simulink model "k1modalprm"  (Simulink 8.6)
settings: Solver=VariableStepAuto  StartTime=0.0  StopTime=10.0  RelTol=1e-3
libraries: cdsIPCx x18, cdsAdcx0 x1, VISMODAL_MASTER x1, cdsParameters x1
settings Model: Creator=controls  LastModifiedBy=controls
settings DataIOCC: SaveFormat=Dataset  SignalLoggingSaveFormat=Dataset
settings OptimizationCC: ExpressionDepthLimit=128
settings DebuggingCC: UnderspecifiedInitializationDetection=Simplified  MergeDetectMultiDrivingBlocksExec=error  SolverPrmCheckMsg=none  FcnCallInpInsideContextMsg=EnableAllAsError  StateNameClashWarn=none
settings HardwareCC: ProdBitPerPointer=64  ProdLargestAtomicFloat=Float  ProdIntDivRoundTo=Zero  ProdEndianess=LittleEndian  ProdWordSize=64  ProdHWDeviceType=Intel->x86-64 (Windows64)
settings GRTTargetCC: GeneratePreprocessorConditionals=Use local settings  CombineOutputUpdateFcns=on  GRTInterface=off
settings ConfigComp: CovModelRefEnable=off

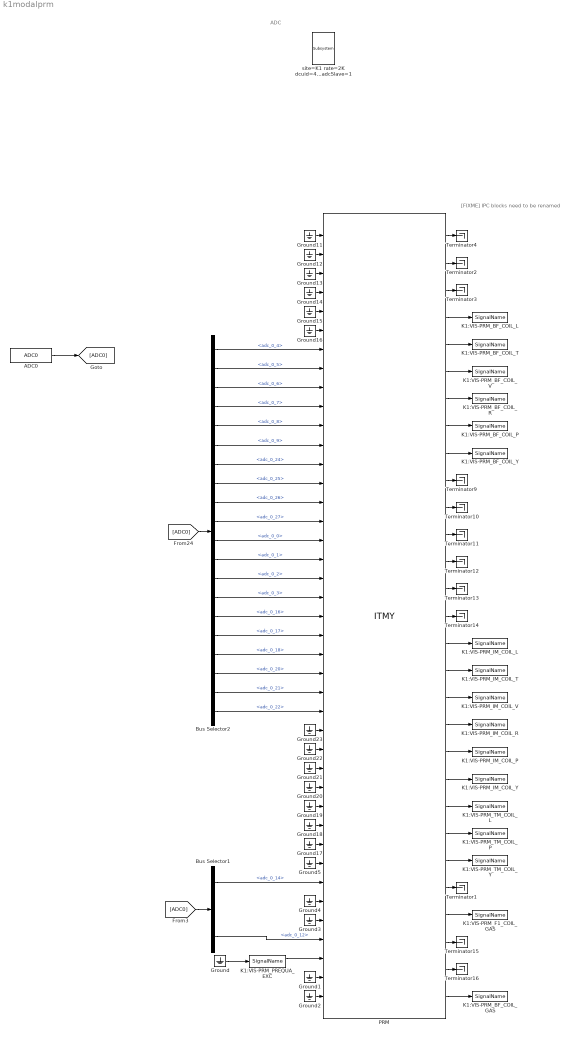
== system k1modalprm ==
  note: ADC
  note: [FIXME] IPC blocks need to be renamed
  ADC0 : cdsAdcx0/ADC0  Tag=cdsAdc  Description=|
      | type-GSC_16AI64SSA
      | card_num=0
      settings: AttributesFormatString=%<Description>\n%<Tag>
  Bus Selector1 : BusSelector  Description=ADC Selector  OutputSignals=adc_0_14,adc_0_13,adc_0_12
      settings: AttributesFormatString=%<Description>
  Bus Selector2 : BusSelector  Description=ADC Selector  OutputSignals=adc_0_4,adc_0_5,adc_0_6,adc_0_7,adc_0_8,adc_0_9,adc_0_24,adc_0_25,adc_0_26,adc_0_27,adc_0_0,adc_0_1,adc_0_2,adc_0_3,adc_0_16,adc_0_17,adc_0_18,adc_0_20,adc_0_21,adc_0_22
      settings: AttributesFormatString=%<Description>
  Ground{,1..5,11..23} (19 alike) : Ground
  K1:VIS-PRM_BF_COIL_GAS : cdsIPCx/SignalName  Tag=cdsIPCx_SHMEM  Description=Inter-Process Communication via Shared memory.
      settings: AttributesFormatString=%<Tag>
  K1:VIS-PRM_BF_COIL_L : cdsIPCx/SignalName  Tag=cdsIPCx_SHMEM  Description=Inter-Process Communication via Shared memory.
      settings: AttributesFormatString=%<Tag>
  K1:VIS-PRM_BF_COIL_P : cdsIPCx/SignalName  Tag=cdsIPCx_SHMEM  Description=Inter-Process Communication via Shared memory.
      settings: AttributesFormatString=%<Tag>
  K1:VIS-PRM_BF_COIL_R : cdsIPCx/SignalName  Tag=cdsIPCx_SHMEM  Description=Inter-Process Communication via Shared memory.
      settings: AttributesFormatString=%<Tag>
  K1:VIS-PRM_BF_COIL_T : cdsIPCx/SignalName  Tag=cdsIPCx_SHMEM  Description=Inter-Process Communication via Shared memory.
      settings: AttributesFormatString=%<Tag>
  K1:VIS-PRM_BF_COIL_V : cdsIPCx/SignalName  Tag=cdsIPCx_SHMEM  Description=Inter-Process Communication via Shared memory.
      settings: AttributesFormatString=%<Tag>
  K1:VIS-PRM_BF_COIL_Y : cdsIPCx/SignalName  Tag=cdsIPCx_SHMEM  Description=Inter-Process Communication via Shared memory.
      settings: AttributesFormatString=%<Tag>
  K1:VIS-PRM_F1_COIL_GAS : cdsIPCx/SignalName  Tag=cdsIPCx_SHMEM  Description=Inter-Process Communication via Shared memory.
      settings: AttributesFormatString=%<Tag>
  K1:VIS-PRM_IM_COIL_L : cdsIPCx/SignalName  Tag=cdsIPCx_SHMEM  Description=Inter-Process Communication via Shared memory.
      settings: AttributesFormatString=%<Tag>
  K1:VIS-PRM_IM_COIL_P : cdsIPCx/SignalName  Tag=cdsIPCx_SHMEM  Description=Inter-Process Communication via Shared memory.
      settings: AttributesFormatString=%<Tag>
  K1:VIS-PRM_IM_COIL_R : cdsIPCx/SignalName  Tag=cdsIPCx_SHMEM  Description=Inter-Process Communication via Shared memory.
      settings: AttributesFormatString=%<Tag>
  K1:VIS-PRM_IM_COIL_T : cdsIPCx/SignalName  Tag=cdsIPCx_SHMEM  Description=Inter-Process Communication via Shared memory.
      settings: AttributesFormatString=%<Tag>
  K1:VIS-PRM_IM_COIL_V : cdsIPCx/SignalName  Tag=cdsIPCx_SHMEM  Description=Inter-Process Communication via Shared memory.
      settings: AttributesFormatString=%<Tag>
  K1:VIS-PRM_IM_COIL_Y : cdsIPCx/SignalName  Tag=cdsIPCx_SHMEM  Description=Inter-Process Communication via Shared memory.
      settings: AttributesFormatString=%<Tag>
  K1:VIS-PRM_PREQUA_EXC : cdsIPCx/SignalName  Tag=cdsIPCx_SHMEM  Description=Inter-Process Communication via Shared memory.
      settings: AttributesFormatString=%<Tag>
  K1:VIS-PRM_TM_COIL_L : cdsIPCx/SignalName  Tag=cdsIPCx_SHMEM  Description=Inter-Process Communication via Shared memory.
      settings: AttributesFormatString=%<Tag>
  K1:VIS-PRM_TM_COIL_P : cdsIPCx/SignalName  Tag=cdsIPCx_SHMEM  Description=Inter-Process Communication via Shared memory.
      settings: AttributesFormatString=%<Tag>
  K1:VIS-PRM_TM_COIL_Y : cdsIPCx/SignalName  Tag=cdsIPCx_SHMEM  Description=Inter-Process Communication via Shared memory.
      settings: AttributesFormatString=%<Tag>
  PRM : VISMODAL_MASTER/ITMY
  Terminator{1..4,9..16} (12 alike) : Terminator
  site=K1 rate=2K dcuid=45 host=k1prm specific_cpu=3 adcSlave=1 : cdsParameters/Subsystem  Tag=cdsParameters  Description=|
      | Purpose:                                                                                                                                                                                                                                
      | Provide system parameters to the FE code generator to properly configure the generated EPICS names, rep rate of the FE controller, and the Data Acquisition node ID for proper storage of data from this FE controller.                 
      |                                                                                                                                                                                                                                         
      | Useage:                                                                                                                                                                                                                                 
      | The part NAME field is used to identify the FE parameters. It must be of the form:                                                                                                                                                      
      | site=                                                                                                                                                                                                                                   
      | rate=                                                                                                                                                                                                                                   
      | dcuid=                                                                                                                                                                                                                                  
      |                                                                                                                                                                                                                                         
      | Where:                                                                                                                                                                                                                                  
      | site= argument may be H1, H2, L1, M1, G1, either as a single argument or multiple, for example site=H1,H2. These are the only names allowed. These will become the first two characters of all EPICS and signal names (for example G1:).
      |                                                                                                                                                                                                                                         
      | rate= may be 2K, 16K, 32K, or 64K                                                                                                                                                                                                       
      |                                                                                                                                                                                                                                         
      | dcuid= is site specific ie it must be unique at each site.
      settings: AttributesFormatString=%<Tag>
  wires:
  PRM/16 -> K1:VIS-PRM_IM_COIL_L/1
  PRM/17 -> K1:VIS-PRM_IM_COIL_T/1
  PRM/18 -> K1:VIS-PRM_IM_COIL_V/1
  PRM/19 -> K1:VIS-PRM_IM_COIL_R/1
  PRM/20 -> K1:VIS-PRM_IM_COIL_P/1
  PRM/21 -> K1:VIS-PRM_IM_COIL_Y/1
  PRM/22 -> K1:VIS-PRM_TM_COIL_L/1
  PRM/23 -> K1:VIS-PRM_TM_COIL_P/1
  PRM/24 -> K1:VIS-PRM_TM_COIL_Y/1
  PRM/1 -> Terminator4/1
  PRM/2 -> Terminator2/1
  PRM/3 -> Terminator3/1
  PRM/26 -> K1:VIS-PRM_F1_COIL_GAS/1
  PRM/29 -> K1:VIS-PRM_BF_COIL_GAS/1
  K1:VIS-PRM_PREQUA_EXC/1 -> PRM/39
  Ground/1 -> K1:VIS-PRM_PREQUA_EXC/1
  Ground1/1 -> PRM/40
  Ground2/1 -> PRM/41
  ADC0/1 -> [ADC0]
  [ADC0] -> Bus Selector2/1
  Bus Selector2/7 -> PRM/13  "<adc_0_24>"
  Bus Selector2/8 -> PRM/14  "<adc_0_25>"
  Bus Selector2/9 -> PRM/15  "<adc_0_26>"
  Bus Selector2/10 -> PRM/16  "<adc_0_27>"
  Bus Selector2/11 -> PRM/17  "<adc_0_0>"
  Bus Selector2/12 -> PRM/18  "<adc_0_1>"
  Bus Selector2/13 -> PRM/19  "<adc_0_2>"
  Bus Selector2/14 -> PRM/20  "<adc_0_3>"
  [ADC0] -> Bus Selector1/1
  Bus Selector1/3 -> PRM/38  "<adc_0_12>"
  Ground3/1 -> PRM/37
  Ground4/1 -> PRM/36
  Ground11/1 -> PRM/1
  Ground12/1 -> PRM/2
  Ground13/1 -> PRM/3
  Ground14/1 -> PRM/4
  Ground15/1 -> PRM/5
  Ground16/1 -> PRM/6
  Ground17/1 -> PRM/33
  Ground18/1 -> PRM/32
  Ground19/1 -> PRM/31
  Ground20/1 -> PRM/30
  PRM/10 -> Terminator9/1
  PRM/11 -> Terminator10/1
  PRM/12 -> Terminator11/1
  PRM/13 -> Terminator12/1
  PRM/14 -> Terminator13/1
  PRM/15 -> Terminator14/1
  PRM/27 -> Terminator15/1
  PRM/28 -> Terminator16/1
  Ground21/1 -> PRM/29
  Ground22/1 -> PRM/28
  Ground23/1 -> PRM/27
  Bus Selector2/15 -> PRM/21  "<adc_0_16>"
  Bus Selector2/1 -> PRM/7  "<adc_0_4>"
  Bus Selector2/2 -> PRM/8  "<adc_0_5>"
  Bus Selector2/3 -> PRM/9  "<adc_0_6>"
  Bus Selector2/4 -> PRM/10  "<adc_0_7>"
  Bus Selector2/5 -> PRM/11  "<adc_0_8>"
  Bus Selector2/6 -> PRM/12  "<adc_0_9>"
  Bus Selector2/16 -> PRM/22  "<adc_0_17>"
  Bus Selector2/17 -> PRM/23  "<adc_0_18>"
  Bus Selector2/20 -> PRM/26  "<adc_0_22>"
  Bus Selector2/19 -> PRM/25  "<adc_0_21>"
  Bus Selector2/18 -> PRM/24  "<adc_0_20>"
  Bus Selector1/1 -> PRM/35  "<adc_0_14>"
  Ground5/1 -> PRM/34
  PRM/25 -> Terminator1/1
  PRM/4 -> K1:VIS-PRM_BF_COIL_L/1
  PRM/5 -> K1:VIS-PRM_BF_COIL_T/1
  PRM/6 -> K1:VIS-PRM_BF_COIL_V/1
  PRM/7 -> K1:VIS-PRM_BF_COIL_R/1
  PRM/8 -> K1:VIS-PRM_BF_COIL_P/1
  PRM/9 -> K1:VIS-PRM_BF_COIL_Y/1
